simulink model "airgk"  (Simulink 8.7)
settings: Solver=ode45  StartTime=0  StopTime=250  RelTol=1e-3
undefined symbols (not defined in the file or in its folder): GM1, x0, xfix
undefined symbols (not defined in the file): AM, GM2
libraries: airlib x1
(part 1 of 2)
settings Model: Creator=kumabhi  LastModifiedBy=kumabhi
settings DataIOCC: LimitDataPoints=off  SignalLoggingSaveFormat=ModelDataLogs  SaveOutput=off  SaveTime=off
settings OptimizationCC: BlockReduction=off  BooleanDataType=off  InitFltsAndDblsToZero=on
settings DebuggingCC: SaveWithParameterizedLinksMsg=none  SignalResolutionControl=TryResolveAllWithWarning  MultiTaskDSMMsg=warning  MultiTaskCondExecSysMsg=none  StrictBusMsg=None
settings HardwareCC: ProdBitPerPointer=64  ProdLargestAtomicFloat=Float  ProdIntDivRoundTo=Zero  ProdEndianess=LittleEndian  ProdWordSize=64  ProdHWDeviceType=Intel->x86-64 (Windows64)  TargetUnknown=on
settings GRTTargetCC: TargetFcnLib=ansi_tfl_tmw.mat  GeneratePreprocessorConditionals=Use local settings  CombineOutputUpdateFcns=off  GRTInterface=on
settings ConfigComp: CovModelRefEnable=off

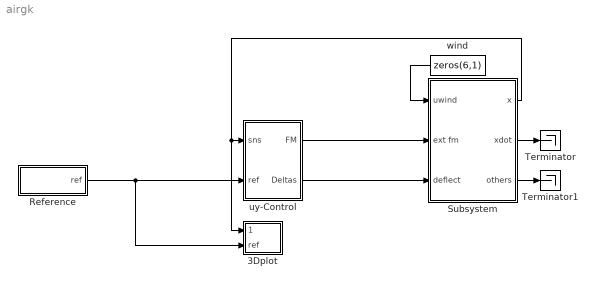
== system airgk ==
  3Dplot : Subsystem
  Reference : Subsystem  mask(Reference Path Generation){Px=[0          2000          2000             0             0             0], Py=[0             0          2000          2000          1000             0], Ph=[60           100            60           500            60            60], Pt=[0   33.3400   66.6800  100.8105  119.0191  135.6858], T=0.05}
      mask prompts: Px "X Positions"; Py "Y Positions"; Ph "H Positions"; Pt "Time"; T "Sample Time"
      mask help: This block generates a 3D trajectory. The output is a vector containing the position and velocity of a point that sequentially visits each X,Y,Z position at the corresponding time. The velocity is constant between one visited point and the next.
      mask Help: This block generates a 3D trajectory. The output is a vector containing the position and velocity of a point that sequentially visits each X,Y,Z position at the corresponding time. The velocity is constant between one visited point and the next.
  Subsystem : Subsystem
  Terminator : Terminator
  Terminator1 : Terminator
  uy-Control : Subsystem  mask(General Nonlinear Aircraft Controller){GM1=[0.5486  5.1511  2.8261   47.2259  90.9483  111.4754   0  -6.6462  0   190.512], CD_wind=[0.060  0.430  0  0.0180  0], CL_wind=[0.385  4.78  8.05  0.401  0], Cm_body=[0.194  -2.12   -36.6   -1.76    0], Cl_body=[0   -0.023   -0.450   0.265   -0.161  -0.00229], Cn_body=[0    0.109  -0.110  -0.200    0.0200  -0.0917], K=[-6.75 9 -9 13.5 0.3], THor=15, Ts=0.05}
      mask prompts: GM1 "Geometry and Mass : [cbar   b    S    Ix   Iy   Iz   Jxy  Jxz  Jyz  m]"; CD_wind "Aerodynamic D-Force Derivatives : [CD0 CDa CDq CDde CDih]"; CL_wind "Aerodynamic L-Force Derivatives : [CL0 CLa CLq CLde CLih]"; Cm_body "Aerodynamic Y-Moment Derivatives : [Cm0 Cma Cmq Cmde Cmih]"; Cl_body "Aerodynamic X-moment Derivatives : [Cl0 Clb Clp Clr Clda Cldr]"; Cn_body "Aerodynamic Z-moment Derivatives : [Cn0 Cnb Cnp Cnr Cnda Cndr]"; K "Controller Coefficients: [Ka Kb Kc Kd Ku]"; THor "Horizon Time"; Ts "Sampling Time"
      mask help:
      | This block is a general feedback linearization controller for aircraft.
      | The first input is a vector contains the 12 aircraft states.
      | The second input contains the reference position and velocity.
      | The output contains the commanded deflections (elevator, aileron and rudder) and the thrust force along the body x axis. Geometry, Mass and Aerodynamic Derivatives should match the ones of the aircraft to be controlled. Ka,Kb,Kc,Kd, are the state space (scalar) coefficients of a PID controller for the feedback linearized attitude dynamics, which behaves as a double integrator system. Ku is the proportional forward velocity controller. The Horizon time is the approximated time lag between reference and actual trajectory. Usually only the aircraft related coefficients need to be changed when applying the controller to a different aircraft.
      mask Help:
      | <p>
      |   This block is a general feedback linearization controller for aircraft.
      |   The first input is a vector contains the 12 aircraft states.
      |   The second input contains the reference position and velocity.
      |   The output contains the commanded deflections (elevator,
      |   aileron and rudder) and the thrust force along the body x axis.
      |   Geometry, Mass and Aerodynamic Derivatives should match the
      |   ones of the aircraft to be controlled. Ka,Kb,Kc,Kd, are the state space
      |   (scalar) coefficients of a PID controller for the feedback linearized
      |   attitude dynamics, which behaves as a double integrator system.
      |   Ku is the proportional forward velocity controller. The Horizon time
      |   is the approximated time lag between reference and actual trajectory.
      |   Usually only the aircraft related coefficients need to be changed
      |   when applying the controller to a different aircraft.
      | </p>
      | <p>
      | Note that neither flaps nor stabilators can be used by this control. Also, this control can be used only when the linearized system having thrust, elevators, ailerons, rudder as inputs, and speed, roll, pitch, yaw as outputs is non-minimum phase. Usually such a system has 2 zeros on the negative real axis, related to alpha and beta respectively. Only occasionally the zero related to beta is on the positive real axis. In those cases the system is non-minimum phase and this controller is not usable anymore.
      | </p>
      | <p>
      | The control surface sign conventions are the same adopted in books such as Stevens-Lewis and Etkin, and in many flight simulators,
      | including the FDC toolbox. <br>
      | Specifically, positive elevator deflection causes negative pitching moment (Cmde &#60 0), positive rudder deflection causes negative yawing
      | moment (Cndr &#60 0), and positive aileron deflection causes negative rolling moment (Clda &#60 0). Another way to say the same thing is
      | that, the positive elevators deflection is Trailing Edge Down (TED), the positive rudder(s) deflection is Trailing Edge Left (TEL), and,
      | taking as TED the positive ailerons deflection, da=K*(da_right-da_left), with K usually equal to 1 (FDC) or 1/2.
      | </p>
      | <p>
      | Since this block is largely based on the FDC toolbox, i redirect you to the FDC Toolbox manual, for a good explanation of the underlying
      | components. Besides the mask and the fact that the aerodynamic derivatives are expressed in the stability axis, the only relevant difference
      | with the FDC toolbox is that in the computation of the aerodynamic forces, q is normalized as q*cbar/2V instead of q*cbar/V. The majority
      | of aeronautics books that i've seen use q*cbar/2V.
      | </p>
      | <p>
      | Please note that the International Measurement System is adopted. So, lengths are in meters, masses in Kg, and inertia moments in Kg*m^2.
      | Moreover, forces are in N, moments in N*m, accelerations in g, and angles in radians. For those that use the english system, here are some useful
      | conversion factors: <br>
      | 1 ft   = 0.3048 m, 1 lb   = 0.4536 Kg, 1 slug = 14.593903 Kg ,  1 slug*ft^2 = 1.355818 Kg*m^2
      | <br>
      | </p>
      | <p>
      | Finally, there is an <A HREF="http://www.aae.uiuc.edu/m-selig/apasim/Aircraft-uiuc.html">excellent source</A> of aircraft aerodynamic data
      | which is mantained by Michael S. Selig, Rob Deters, and Glen Dimock at the university of Urbana-Champaign. To use any of the given models
      | you just need to type the supplied aircraft data in the block mask.
      | </p>
      | <p>
      | <p>
      | July 2006, Giampiero Campa
      | </p>
      | </p>
      mask Display: disp('General\nAircraft\nController')
  wind : Constant  Value=zeros(6,1)
  wires:
  wind/1 -> Subsystem/1(" uwind")
  Reference/1(ref) -> uy-Control/2(ref), 3Dplot/2(ref)
  uy-Control/1(FM) -> Subsystem/2(ext fm)
  uy-Control/2(Deltas) -> Subsystem/3(deflect)
  Subsystem/1(x) -> 3Dplot/1(meas), uy-Control/1(sns)
  Subsystem/2(xdot) -> Terminator/1
  Subsystem/3(others) -> Terminator1/1

== system airgk/3Dplot ==
  note: Set Camera position to [0 0 1] for 2D view
  meas : Inport
  ref : Inport  Port=2
  3D Graph : S-Function  LoadFcn=if exist('sfun3d','file'), sfun3d([],[],[],'LoadBlock'); end  FunctionName=sfun3d  Parameters=ax,T,np,cp,gd,ls,mk,mx,hd,tb  SFunctionDeploymentMode=off  EnableBusSupport=off  mask(3D Graph){np=2, ax=[-1 3 -1 3 0 0.5]*1e3, mx=1e3, T=0.1, cp=[-10 -20 3]*1e3, gd=on, hd=on, tb=off, ls=-, mk=none}
      mask prompts: np "Number of moving points (lines)"; ax "Range: [xmin xmax  ymin ymax zmin zmax]"; mx "Max number of points in each line"; T "Sampling Time"; cp "Camera position (use [0 0 1] for 2D XY view)"; gd "Grid (on|off)"; hd "HeadMarkers (on|off)"; tb "Toolbar (on|off)"; ls "LineStyle"; mk "LineMarker"
      mask help:
      | This block plots the position of several points in the XYZ space. The input contains the coordinates of all the points (x1,y1,z1,x2,y2,z2,...).
      | The number of moving points (lines), the XYZ ranges, sampling time, camera position, and grid (among other things) can be set as mask parameters.
      settings: CopyFcn=if exist('sfun3d','file'), sfun3d([],[],[],'CopyBlock'); end  DeleteFcn=if exist('sfun3d','file'), sfun3d([],[],[],'DeleteBlock'); end  NameChangeFcn=if exist('sfun3d','file'), sfun3d([],[],[],'NameChange'); end
      mask Help:
      | This block plots the position of several points in the XYZ space. The input contains the coordinates of all the points (x1,y1,z1,x2,y2,z2,...).
      | The number of moving points (lines), the XYZ ranges, sampling time, camera position, and grid (among other things) can be set as mask parameters.
      mask TypeOptions ls: - | -- | : | -. | none
      mask TypeOptions mk: none | . | + | o | * | x | square | diamond | v | ^ | > | < | pentagram | hexagram
      mask Display: plot([.05 .95 .95 .05 .05],[.45 .45 .95 .95 .45], 0.5+cos(0:0.1:2*pi)*0.3,0.7+sin(0:0.1:2*pi)*0.2)
  Mux3 : Mux  Inputs=[3 3]
  real xyz : Selector  InputPortWidth=12  IndexOptions=Index vector (dialog)  Indices=10:12  OutputSizes=1
  ref xyz : Selector  InputPortWidth=6  IndexOptions=Index vector (dialog)  Indices=1:3  OutputSizes=1
  wires:
  real xyz/1 -> Mux3/1
  ref/1 -> ref xyz/1
  meas/1 -> real xyz/1
  ref xyz/1 -> Mux3/2
  Mux3/1 -> 3D Graph/1

== system airgk/Reference ==
  Clock : Clock
  Delay : UnitDelay  InitialCondition=[Px(1) Py(1) Ph(1)]  SampleTime=T
  Derivative : Subsystem  mask(Time Derivative){x0=[Px(1) Py(1) Ph(1)]'-[Px(2)-Px(1) Py(2)-Py(1) Ph(2)-Ph(1)]'/(Pt(2)-Pt(1))*T, T=T}
      mask prompts: x0 "Initial Condition"; T "Sampling Time"
      mask help:
      | First order approximation of the time derivative of the input signal,
      |   the original one is buggy.
  Hd(t) : Lookup  InputValues=Pt  Table=Ph  SaturateOnIntegerOverflow=on
  Horizon Time : Constant  Value=0
  Math Function : Math  Operator=mod  SaturateOnIntegerOverflow=on
  Mux : Mux  Inputs=3
  Mux2 : Mux  Inputs=[3 3]
  Sum2 : Sum  Inputs=++|  SaturateOnIntegerOverflow=on  InputSameDT=on  OutDataTypeStr=Inherit: Same as first input
  Time Limit : Constant  Value=Pt(end)
  Xd(t) : Lookup  InputValues=Pt  Table=Px  SaturateOnIntegerOverflow=on
  Yd(t) : Lookup  InputValues=Pt  Table=Py  SaturateOnIntegerOverflow=on
  ref : Outport
  wires:
  Mux/1 -> Derivative/1(x), Delay/1
  Time Limit/1 -> Math Function/2
  Math Function/1 -> Hd(t)/1, Yd(t)/1, Xd(t)/1
  Clock/1 -> Sum2/2
  Horizon Time/1 -> Sum2/1
  Sum2/1 -> Math Function/1
  Hd(t)/1 -> Mux/3
  Yd(t)/1 -> Mux/2
  Xd(t)/1 -> Mux/1
  Delay/1 -> Mux2/1
  Derivative/1(xdot) -> Mux2/2
  Mux2/1 -> ref/1

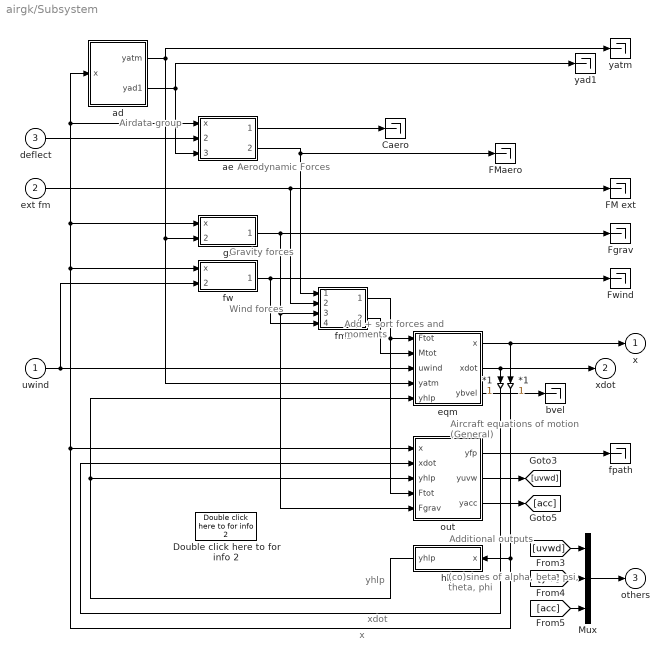
== system airgk/Subsystem ==
  note: xdot
  note: x
  note: yhlp
  note: Additional outputs
  note: Aircraft equations
      | of motion (General)
  note: Wind forces
  note: Gravity forces
  note: Aerodynamic
      | Forces
  note: (co)sines of
      | alpha, beta,
      | psi, theta, phi
  note: Add + sort
      | forces and
      | moments
  note: Airdata group
  " uwind" : Inport
  ext fm : Inport  Port=2
  deflect : Inport  Port=3
  " *1" : Gain  SaturateOnIntegerOverflow=on  OutDataTypeStr=Inherit: Same as input  ParamDataTypeStr=Inherit: Same as input
  *1 : Gain  SaturateOnIntegerOverflow=on  OutDataTypeStr=Inherit: Same as input  ParamDataTypeStr=Inherit: Same as input
  Caero : Terminator
  Double click here to for info 2 : airlib/DT-B747/Double click here to for info 2  SystemSampleTime=-1
  FM ext : Terminator
  FMaero : Terminator
  Fgrav : Terminator
  Fwind : Terminator
  Mux : Mux  Inputs=[3 3 6]
  ad : Subsystem
  ae : Subsystem
  bvel : Terminator
  eqm : Subsystem
  fms : Subsystem  mask(FMsort){}
      mask help: Forces and Moments sorting block
      mask Display: disp('FMsort')
  fpath : Terminator
  fw : Subsystem  mask(fwind){m=GM1(10)}
      mask prompts: m "Mass of the aircraft [kg]:"
      mask help: Forces due to non-steady atmosphere.
      mask Display: disp('Fwind')
  gr : Subsystem  mask(Gravity){m=GM1(10)}
      mask prompts: m "Mass of the aircraft [kg]:"
      mask help: Gravity forces.
      mask Display: disp('Gravity')
  hlp : Subsystem  mask(Hlpfcn){}
      mask help: Help sines and cosines
      mask Display: disp('hlpfcn')
  out : Subsystem
  yad1 : Terminator
  yatm : Terminator
  x : Outport
  xdot : Outport  Port=2
  others : Outport  Port=3
  wires:
  fms/1(Ftot) -> out/4(Ftot), eqm/1(Ftot)
  ext fm/1 -> fms/2(FMprop), FM ext/1
  deflect/1 -> ae/2(uaero)
  ae/1(Caero) -> Caero/1
  eqm/3(ybvel) -> bvel/1
  out/1(yfp) -> fpath/1
  ad/2(yad1) -> yad1/1, ae/3(yad1)
  ad/1(yatm) -> yatm/1, eqm/4(yatm), gr/2(yatm)
  out/3(yacc) -> [acc]
  fw/1(Fwind) -> Fwind/1, fms/4(Fwind)
  ae/2(FMaero) -> FMaero/1, fms/1(FMaero)
  hlp/1(yhlp) -> eqm/5(yhlp), out/3(yhlp)
  " uwind"/1 -> eqm/3(uwind), fw/2(uwind)
  *1/1 -> out/2(xdot)
  gr/1(Fgrav) -> fms/3(Fgrav), out/5(Fgrav), Fgrav/1
  " *1"/1 -> hlp/1(x), out/1(x), fw/1(x), gr/1(x), ae/1(x), ad/1(x)
  eqm/2(xdot) -> xdot/1, *1/1
  eqm/1(x) -> x/1, " *1"/1
  fms/2(Mtot) -> eqm/2(Mtot)
  out/2(yuvw) -> [uvwd]
  [uvwd] -> Mux/1
  [ydl] -> Mux/2
  [acc] -> Mux/3
  Mux/1 -> others/1

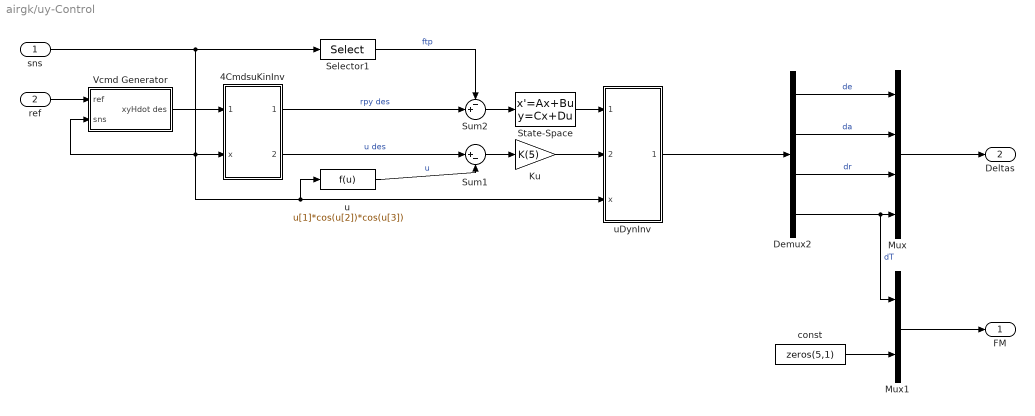
== system airgk/uy-Control ==
  sns : Inport
  ref : Inport  Port=2
  4CmdsuKinInv : Subsystem  mask(Inverse Nonlinear Aircraft Model){Psi0=0, T=Ts}
      mask prompts: Psi0 "Initial Psi (used for Turn Coordination Derivative)"; T "Sampling Time (used for Turn Coordination Derivative)"
      mask help:
      | This block uses an exact turn coordination constraint
      |   to obtain velocity and attitude commands from desired accelerations.
      |   The first input contains the desired derivatives of the position (x,y,H).
      |   The second input contains the actual state of the aircraft.
      |   The first and second outputs contain respectively the commanded
      |   euler angles and the speed along the x axis (u=Vcos(a)cos(b)).
      |   NB : The International measurement system (MKS) is adopted.
      mask Help:
      | This block uses an exact turn coordination constraint
      |   to obtain velocity and attitude commands from desired accelerations.
      |   The first input contains the desired derivatives of the position (x,y,H).
      |   The second input contains the actual state of the aircraft.
      |   The first and second outputs contain respectively the commanded
      |   euler angles and the speed along the x axis (u=Vcos(a)cos(b)).
      |   NB : The International measurement system (MKS) is adopted.
      mask Display: disp('u-Inverse\nKinematic\nModel')
  Demux2 : Demux
  Ku : Gain  Gain=K(5)  SaturateOnIntegerOverflow=on  OutDataTypeStr=Inherit: Same as input  ParamDataTypeStr=Inherit: Same as input
  Mux : Mux  Inputs=[1 1 1 1]
  Mux1 : Mux  Inputs=[1 5]
  Selector1 : Selector  InputPortWidth=12  IndexOptions=Index vector (dialog)  Indices=[9 8 7]  OutputSizes=1
  State-Space : StateSpace  A=K(1)*eye(3)  B=K(2)*eye(3)  C=K(3)*eye(3)  D=K(4)*eye(3)  X0=0
  Sum1 : Sum  Inputs=|+-  SaturateOnIntegerOverflow=on  InputSameDT=on  OutDataTypeStr=Inherit: Same as first input
  Sum2 : Sum  Inputs=-+|  SaturateOnIntegerOverflow=on  InputSameDT=on  OutDataTypeStr=Inherit: Same as first input
  Vcmd Generator : Subsystem  mask(Velocity Command Generator){Kp=1, Kv=0, THor=THor, T=Ts}
      mask prompts: Kp "Position Error Gain"; Kv "Velocity Error Gain"; THor "Horizon Time"; T "Sample Time"
      mask help:
      | The first input is a reference position and velocity vector,
      |   the second one is a current position and velocity vector.
      |   The output is a filtered command in xyHdot .
      mask Help:
      | The first input is a reference position and velocity vector,
      |   the second one is a current position and velocity vector.
      |   The output is a filtered command in xyHdot .
  const : Constant  Value=zeros(5,1)
  u : Fcn  Expr=u[1]*cos(u[2])*cos(u[3])
  uDynInv : Subsystem  mask(Inverse Nonlinear Aircraft Model){GM1=GM1, CD_wind=CD_wind, CL_wind=CL_wind, Cm_body=Cm_body, Cl_body=Cl_body, Cn_body=Cn_body}
      mask prompts: GM1 "Geometry, Mass : [cbar   b    S    Ix   Iy   Iz   Jxy  Jxz  Jyz  m]"; CD_wind "Aerodynamic D-Force Derivatives : [CD0 CDa CDq CDde CDih]"; CL_wind "Aerodynamic L-Force Derivatives : [CL0 CLa CLq CLde CLih]"; Cm_body "Aerodynamic Y-Moment Derivatives : [Cm0 Cma Cmq Cmde Cmih]"; Cl_body "Aerodynamic X-moment Derivatives : [Cl0 Clb Clp Clr Clda Cldr]"; Cn_body "Aerodynamic Z-moment Derivatives : [Cn0 Cnb Cnp Cnr Cnda Cndr]"
      mask help:
      | The first and second inputs contain the desired double derivatives
      |   of the attitude (roll, pitch, and yaw) and the desired detivative of
      |   u=V*cos(alpha)*cos(beta), which is the speed along the x body axis.
      |   The third input contains the actual state of the aircraft.
      |   The output contains the commanded deflections (elevator,
      |   aileron and rudder) and thrust force along the body x axis.
      |   NB : The International measurement system (MKS) is adopted.
      mask init:
      | AM=zeros(6,19);
      | AM(1,[1 2 9 11 12])=reshape(CD_wind,1,5);
      | AM(3,[1 2 9 11 12])=reshape(CL_wind,1,5);
      | AM(5,[1 2 9 11 12])=reshape(Cm_body,1,5);
      | AM(4,[1 5 8 10 13 14])=reshape(Cl_body,1,6);
      | AM(6,[1 5 8 10 13 14])=reshape(Cn_body,1,6);
      | 
      | Ix=GM1(4);Iy=GM1(5);Iz=GM1(6);
      | Jxy=GM1(7);Jxz=GM1(8);Jyz=GM1(9);
      | 
      | detI = Ix*Iy*Iz - 2*Jxy*Jxz*Jyz - Ix*Jyz^2 - Iy*Jxz^2 - Iz*Jxy^2;
      | I1   = Iy*Iz - Jyz^2;I2   = Jxy*Iz + Jyz*Jxz;
      | I3   = Jxy*Jyz + Iy*Jxz;I4   = Ix*Iz - Jxz^2;
      | I5   = Ix*Jyz + Jxy*Jxz;I6   = Ix*Iy - Jxy^2;
      | 
      | Pl  = I1/detI; Pm = I2/detI; Pn = I3/detI;
      | Ppp = -(Jxz*I2 - Jxy*I3)/detI;Ppq = (Jxz*I1 - Jyz*I2 - (Iy-Ix)*I3)/detI;
      | Ppr = -(Jxy*I1 + (Ix-Iz)*I2 - Jyz*I3)/detI;Pqq = (Jyz*I1 - Jxy*I3)/detI;
      | Pqr = -((Iz-Iy)*I1 - Jxy*I2 + Jxz*I3)/detI;Prr = -(Jyz*I1 - Jxz*I2)/detI;
      | 
      | Ql  = I2/detI; Qm = I4/detI; Qn = I5/detI;
      | Qpp = -(Jxz*I4 - Jxy*I5)/detI;Qpq = (Jxz*I2 - Jyz*I4 - (Iy-Ix)*I5)/detI;
      | Qpr = -(Jxy*I2 + (Ix-Iz)*I4 - Jyz*I5)/detI;Qqq = (Jyz*I2 - Jxy*I5)/detI;
      | Qqr = -((Iz-Iy)*I2 - Jxy*I4 + Jxz*I5)/detI;Qrr = -(Jyz*I2 - Jxz*I4)/detI;
      | 
      | Rl  = I3/detI; Rm = I5/detI; Rn = I6/detI;
      | Rpp = -(Jxz*I5 - Jxy*I6)/detI;
      | Rpq = (Jxz*I3 - Jyz*I5 - (Iy-Ix)*I6)/detI;
      | Rpr = -(Jxy*I3 + (Ix-Iz)*I5 - Jyz*I6)/detI;
      | Rqq = (Jyz*I3 - Jxy*I6)/detI;
      | Rqr = -((Iz-Iy)*I3 - Jxy*I5 + Jxz*I6)/detI;
      | Rrr = -(Jyz*I3 - Jxz*I5)/detI;
      | 
      | GM2 = [  Pl   Pm   Pn   Ppp  Ppq  Ppr  Pqq  Pqr  Prr ;
      |                Ql  Qm   Qn   Qpp  Qpq  Qpr  Qqq  Qqr  Qrr ;
      |                Rl  Rm   Rn   Rpp  Rpq  Rpr  Rqq  Rqr  Rrr ];
      | 
      | xfix=1;
      mask Help:
      | <p>
      | This block is an inverse nonlinear 6DOF aircraft model, with a very accurate built-in atmosphere model and constant aerodynamic derivatives.
      | The architecture of the block is largely based on the Aircraft block provided by the <A
      | HREF="http://www.mathworks.com/matlabcentral/fileexchange/loadFile.do?objectId=252&objectType=file">FDC toolbox</A> (Marc Rauw, 1993-2000).
      | </p>
      | <p>
      | The geometric and inertal data of the aircraft are entered as parameters in the first row of the mask, sampling time is the last parameter. The other rows contain the non-dimensional aerodynamic derivatives.
      | </p>
      | <p>
      |   The first and second inputs contain the desired double derivatives
      |   of the attitude (roll, pitch, and yaw) and the desired detivative of
      |   u=V*cos(alpha)*cos(beta), which is the speed along the x body axis.
      |   The third input contains the actual state of the aircraft.
      |   The output contains the commanded deflections (elevator,
      |   aileron and rudder) and thrust force along the body x axis.
      | </p>
      | <p>
      | Note that neither flaps nor stabilators can be used by this control.
      | </p>
      | <p>
      | The control surface sign conventions are the same adopted in books such as Stevens-Lewis and Etkin, and in many flight simulators,
      | including the FDC toolbox. <br>
      | Specifically, positive elevator deflection causes negative pitching moment (Cmde &#60 0), positive rudder deflection causes negative yawing
      | moment (Cndr &#60 0), and positive aileron deflection causes negative rolling moment (Clda &#60 0). Another way to say the same thing is
      | that, the positive elevators deflection is Trailing Edge Down (TED), the positive rudder(s) deflection is Trailing Edge Left (TEL), and,
      | taking as TED the positive ailerons deflection, da=K*(da_right-da_left), with K usually equal to 1 (FDC) or 1/2.
      | </p>
      | <p>
      | Since this block is largely based on the FDC toolbox, i redirect you to the FDC Toolbox manual, for a good explanation of the underlying
      | components. Besides the mask and the fact that the aerodynamic derivatives are expressed in the stability axis, the only relevant difference
      | with the FDC toolbox is that in the computation of the aerodynamic forces, q is normalized as q*cbar/2V instead of q*cbar/V. The majority
      | of aeronautics books that i've seen use q*cbar/2V.
      | </p>
      | <p>
      | Please note that the International Measurement System is adopted. So, lengths are in meters, masses in Kg, and inertia moments in Kg*m^2.
      | Moreover, forces are in N, moments in N*m, accelerations in g, and angles in radians. For those that still use the english system, here are some useful
      | conversion factors: <br>
      | 1 ft   = 0.3048 m, 1 lb   = 0.4536 Kg, 1 slug = 14.593903 Kg ,  1 slug*ft^2 = 1.355818 Kg*m^2
      | <br>
      | </p>
      | <p>
      | Finally, there is an <A HREF="http://www.aae.uiuc.edu/m-selig/apasim/Aircraft-uiuc.html">excellent source</A> of aircraft aerodynamic data
      | which is mantained by Michael S. Selig, Rob Deters, and Glen Dimock at the university of Urbana-Champaign. To use any of the given models
      | you just need to type the supplied aircraft data in the block mask.
      | </p>
      | <p>
      | <p>
      | Feb 2004, Giampiero Campa
      | </p>
      | </p>
      mask Display: disp('4 Cmds\nu-Inverse\nAircraft\nModel')
  FM : Outport
  Deltas : Outport  Port=2
  wires:
  ref/1 -> Vcmd Generator/1(ref)
  Vcmd Generator/1(xyHdot des) -> 4CmdsuKinInv/1(pdotdes)
  Sum2/1 -> State-Space/1
  Ku/1 -> uDynInv/2(udotdes)
  State-Space/1 -> uDynInv/1(ftpddotdes)
  sns/1 -> Selector1/1, 4CmdsuKinInv/2(x), Vcmd Generator/2(sns), u/1, uDynInv/3(x)
  Selector1/1 -> Sum2/1  "ftp"
  4CmdsuKinInv/1(rpycmd) -> Sum2/2  "rpy des"
  4CmdsuKinInv/2(ucmd) -> Sum1/1  "u des"
  u/1 -> Sum1/2  "u"
  Sum1/1 -> Ku/1
  Mux/1 -> Deltas/1
  Mux1/1 -> FM/1
  const/1 -> Mux1/2
  Demux2/4 -> Mux1/1, Mux/4  "dT"
  Demux2/3 -> Mux/3  "dr"
  Demux2/2 -> Mux/2  "da"
  Demux2/1 -> Mux/1  "de"
  uDynInv/1(Cmds) -> Demux2/1

== system airgk/Reference/Derivative ==
  x : Inport
  Product2 : Product  Inputs=/*  SaturateOnIntegerOverflow=on  RndMeth=Zero  InputSameDT=on  OutDataTypeStr=Inherit: Same as first input
  Sum4 : Sum  Inputs=|+-  SaturateOnIntegerOverflow=on  InputSameDT=on  OutDataTypeStr=Inherit: Same as first input
  Unit Delay1 : UnitDelay  InitialCondition=x0  SampleTime=T
  Zero-Order Hold1 : ZeroOrderHold  SampleTime=T
  m : Constant  Value=T
  xdot : Outport
  wires:
  Sum4/1 -> Product2/2
  Unit Delay1/1 -> Sum4/2
  Zero-Order Hold1/1 -> Sum4/1, Unit Delay1/1
  m/1 -> Product2/1
  Product2/1 -> xdot/1
  x/1 -> Zero-Order Hold1/1

== system airgk/Subsystem/ad ==
  x : Inport
  ad1 : Subsystem  mask(Airdata1){}
      mask help: Basic airdata variables
      mask Display: disp('Airdata1')
  atm : Subsystem  mask(Atmosph){}
      mask help: Atmosphere variables
      mask Display: disp('Atmosph')
  yatm : Outport
  yad1 : Outport  Port=2
  wires:
  x/1 -> atm/1(x), ad1/1(x)
  atm/1(yatm) -> ad1/2(yatm), yatm/1
  ad1/1(yad1) -> yad1/1

== system airgk/Subsystem/ae ==
  x : Inport
  uaero : Inport  Port=2
  yad1 : Inport  Port=3
  aero : Subsystem  mask(Aeromod){}
      mask help: Aerodynamic model of the DHC-2 'Beaver'.
      mask Display: disp('Aeromod\n(General)')
  dl : Subsystem  mask(Dimless){cbar=GM1(1), b=GM1(2)}
      mask prompts: cbar "Mean aerodynamic chord [m]:"; b "Wing span [m]:"
      mask help: Dimensionless rotational velocities.
      mask Display: disp('Dimless')
  fmdims : Subsystem  mask(FMdims){cbar=GM1(1), b=GM1(2), S=GM1(3)}
      mask prompts: cbar "Mean aerodynamic chord [m]:"; b "Wing span [m]:"; S "Wing surface [m^2]:"
      mask help:
      | Calculate forces and moments from
      | dimensionless derivatives.
      mask Display: disp('FMdims')
  Caero : Outport
  FMaero : Outport  Port=2
  wires:
  aero/1(Caero) -> Caero/1, fmdims/2(Force / moment derivatives)
  dl/1(ydl) -> aero/3(ydl)
  x/1 -> dl/1(x), aero/1(x)
  uaero/1 -> aero/2(uaero)
  yad1/1 -> fmdims/1(yad1)
  fmdims/1(Forces and moments) -> FMaero/1

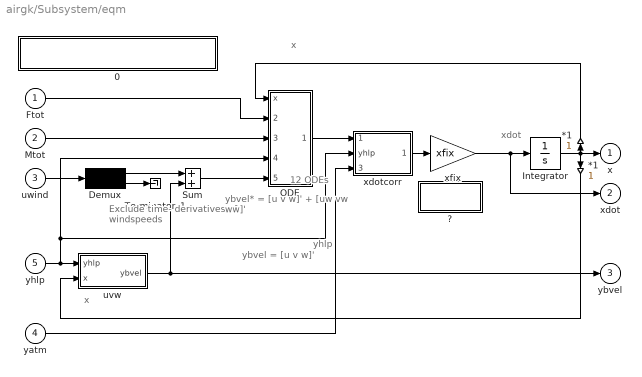
== system airgk/Subsystem/eqm ==
  note: Exclude time-
      | derivatives
      | of windspeeds
  note: ybvel* =
      | [u v w]' +
      | [uw vw ww]'
  note: xdot
  note: x
  note: x
  note: yhlp
  note: ybvel = [u v w]'
  note: 12 ODEs
  Ftot : Inport
  Mtot : Inport  Port=2
  uwind : Inport  Port=3
  yatm : Inport  Port=4
  yhlp : Inport  Port=5
  " *1" : Gain  SaturateOnIntegerOverflow=on  OutDataTypeStr=Inherit: Same as input  ParamDataTypeStr=Inherit: Same as input
  *1 : Gain  SaturateOnIntegerOverflow=on  OutDataTypeStr=Inherit: Same as input  ParamDataTypeStr=Inherit: Same as input
  0 : Subsystem
      mask Display: disp('EQUATIONS OF MOTION (level 3)\nM.O. Rauw')
  "?" : Subsystem
      mask Display: disp('More info\nfor xfix')
  Demux : Demux  Outputs=[3 3]
  Integrator : Integrator  InitialCondition=x0
  ODE : Subsystem
  Sum : Sum  SaturateOnIntegerOverflow=on  InputSameDT=on  OutDataTypeStr=Inherit: Same as first input
  Terminator_1 : Terminator
  uvw : Subsystem  mask(uvw){}
      mask help:
      | Calculation of body-axes velocities
      | u, v, and w
      mask Display: disp('Body-axes\nvelocities')
  xdotcorr : Subsystem  mask(xdotcorr){b=GM1(2), S=GM1(3), m=GM1(10), CYbdot=AM(2,19)}
      mask prompts: b "Wing span [m]:"; S "Wing surface [m^2]:"; m "Mass of the aircraft [kg]:"; CYbdot "Stability-derivative CYbdot:"
      mask help:
      | Correction block to write state
      | equations for DHC-2 Beaver aircraft
      | explicitly.
      mask Display: disp('xdotcorr\n(General)')
  xfix : Gain  Gain=xfix  SaturateOnIntegerOverflow=on  OutDataTypeStr=Inherit: Same as input  ParamDataTypeStr=Inherit: Same as input
  x : Outport
  xdot : Outport  Port=2
  ybvel : Outport  Port=3
  wires:
  Demux/2 -> Terminator_1/1
  yhlp/1 -> uvw/1(yhlp), ODE/4(yhlp), xdotcorr/2(yhlp)
  ODE/1(xdot) -> xdotcorr/1(xdot uncorrected)
  Sum/1 -> ODE/5(ybvel*)
  uvw/1(ybvel) -> ybvel/1, Sum/2
  uwind/1 -> Demux/1
  Demux/1 -> Sum/1
  xdotcorr/1(xdot corrected) -> xfix/1
  yatm/1 -> xdotcorr/3(yatm)
  Ftot/1 -> ODE/2(Ftot)
  Mtot/1 -> ODE/3(Mtot)
  *1/1 -> uvw/2(x)
  Integrator/1 -> x/1, " *1"/1, *1/1
  xfix/1 -> Integrator/1, xdot/1
  " *1"/1 -> ODE/1(x)

== system airgk/Subsystem/fms ==
  FMaero : Inport
  FMprop : Inport  Port=2
  Fgrav : Inport  Port=3
  Fwind : Inport  Port=4
  0 : Subsystem
      mask Display: disp('FMSORT\nM.O. Rauw, October 1997')
  Demux : Demux  Outputs=[3 3]
  Demux1 : Demux  Outputs=[3 3]
  Sum1 : Sum  SaturateOnIntegerOverflow=on  InputSameDT=on  OutDataTypeStr=Inherit: Same as first input
  Sum3 : Sum  Inputs=++++  SaturateOnIntegerOverflow=on  InputSameDT=on  OutDataTypeStr=Inherit: Same as first input
  Ftot : Outport
  Mtot : Outport  Port=2
  wires:
  FMaero/1 -> Demux/1
  FMprop/1 -> Demux1/1
  Demux1/2 -> Sum1/2
  Demux/2 -> Sum1/1
  Fgrav/1 -> Sum3/3
  Demux1/1 -> Sum3/2
  Sum3/1 -> Ftot/1
  Sum1/1 -> Mtot/1
  Demux/1 -> Sum3/1
  Fwind/1 -> Sum3/4

== system airgk/Subsystem/fw ==
  x : Inport
  uwind : Inport  Port=2
  -Xw/m : Fcn  Expr=u[16] + u[5]*u[15] - u[6]*u[14]
  -Yw/m : Fcn  Expr=u[17] - u[4]*u[15] + u[6]*u[13]
  -Zw/m : Fcn  Expr=u[18] + u[4]*u[14] - u[5]*u[13]
  0 : Subsystem
      mask Display: disp('FWIND\nM.O. Rauw, Dec. 1996')
  Mux : Mux  Inputs=3
  Mux1 : Mux  Inputs=[12 6]
  gain : Gain  Gain=-m  SaturateOnIntegerOverflow=on  OutDataTypeStr=Inherit: Same as input  ParamDataTypeStr=Inherit: Same as input
  Fwind : Outport
  wires:
  uwind/1 -> Mux1/2
  x/1 -> Mux1/1
  gain/1 -> Fwind/1
  Mux/1 -> gain/1
  Mux1/1 -> -Yw/m/1, -Zw/m/1, -Xw/m/1
  -Yw/m/1 -> Mux/2
  -Xw/m/1 -> Mux/1
  -Zw/m/1 -> Mux/3

== system airgk/Subsystem/gr ==
  x : Inport
  yatm : Inport  Port=2
  0 : Subsystem
      mask Display: disp('GRAVITY\nM.O. Rauw, October 1997')
  Mux : Mux  Inputs=3
  Mux1 : Mux  Inputs=[12 5]
  Xgr : Fcn  Expr=-m*u[17]*sin(u[8])
  Ygr : Fcn  Expr=m*u[17]*cos(u[8])*sin(u[9])
  Zgr : Fcn  Expr=m*u[17]*cos(u[8])*cos(u[9])
  Fgrav : Outport
  wires:
  Xgr/1 -> Mux/1
  Ygr/1 -> Mux/2
  Mux/1 -> Fgrav/1
  Mux1/1 -> Ygr/1, Xgr/1, Zgr/1
  Zgr/1 -> Mux/3
  x/1 -> Mux1/1
  yatm/1 -> Mux1/2

== system airgk/Subsystem/hlp ==
  x : Inport
  0 : Subsystem
      mask Display: disp('HELP FUNCTIONS\n(often used sines and cosines)\nM.O. Rauw, October 1997')
  Mux : Mux  Inputs=11
  cos alpha : Fcn  Expr=cos(u[2])
  cos beta : Fcn  Expr=cos(u[3])
  cos phi : Fcn  Expr=cos(u[9])
  cos psi : Fcn  Expr=cos(u[7])
  cos theta : Fcn  Expr=cos(u[8])
  sin alpha : Fcn  Expr=sin(u[2])
  sin beta : Fcn  Expr=sin(u[3])
  sin phi : Fcn  Expr=sin(u[9])
  sin psi : Fcn  Expr=sin(u[7])
  sin theta : Fcn  Expr=sin(u[8])
  tan beta : Fcn  Expr=tan(u[3])
  yhlp : Outport
  wires:
  x/1 -> sin psi/1, sin beta/1, cos beta/1, sin alpha/1, cos alpha/1, tan beta/1, sin theta/1, cos theta/1, sin phi/1, cos phi/1, cos psi/1
  cos alpha/1 -> Mux/1
  sin alpha/1 -> Mux/2
  cos beta/1 -> Mux/3
  sin beta/1 -> Mux/4
  tan beta/1 -> Mux/5
  sin psi/1 -> Mux/6
  cos psi/1 -> Mux/7
  sin theta/1 -> Mux/8
  cos theta/1 -> Mux/9
  sin phi/1 -> Mux/10
  Mux/1 -> yhlp/1
  cos phi/1 -> Mux/11

== system airgk/Subsystem/out ==
  note: Flightpath
      | variables
  note: du/dt, dv/dt, dw/dt
      | (output equations!)
  note: Body-axes accelerations
      | and specific forces
  x : Inport
  xdot : Inport  Port=2
  yhlp : Inport  Port=3
  Ftot : Inport  Port=4
  Fgrav : Inport  Port=5
  0 : Subsystem
      mask Display: disp('Additional outputs (level 3)\nM.O. Rauw')
  accel : Subsystem  mask(accel){m=GM1(10)}
      mask prompts: m "Mass of the aircraft [kg]:"
      mask help:
      | Body axes accelerations and
      | specific forces.
      mask Display: disp('Accel')
  fp : Subsystem  mask(Flpath){alpha0=x0(2)}
      mask prompts: alpha0 "Initial value of angle of attack, alpha0:"
      mask help: Flightpath related parameters.
      mask Display: disp('flpath')
  uvwdot : Subsystem  mask(uvwdot){}
      mask help: Calculation of du/dt, dv/dt, and dw/dt.
      mask Display: disp('uvwdot')
  yfp : Outport
  yuvw : Outport  Port=2
  yacc : Outport  Port=3
  wires:
  fp/1(yfp) -> yfp/1
  uvwdot/1(yuvw =  [udot; vdot; wdot]) -> yuvw/1
  yhlp/1 -> uvwdot/3(yhlp)
  Ftot/1 -> accel/1(Ftot)
  accel/1(yacc) -> yacc/1
  xdot/1 -> fp/2(xdot), uvwdot/2(xdot)
  x/1 -> fp/1(x), uvwdot/1(x)
  Fgrav/1 -> accel/2(Fgrav)

== system airgk/uy-Control/4CmdsuKinInv ==
  pdotdes : Inport
  x : Inport  Port=2
  Demux : Demux  Outputs=3
  Exact Turn Coordination : Subsystem
  Mux1 : Mux  Inputs=3
  Mux2 : Mux  Inputs=[3 12]
  a2c  xy : Subsystem  mask(Continuous Atan2 Function){L=4, T=T}
      mask prompts: L "Maximum angular distance covered during the sample time (< 2*pi)"; T "Sample Time"
      mask help:
      | This atan2 does not jump between pi and -pi.
      |   It is assumed that the inputs changes smoothly in time,
      |   specifically it is assumed that the maximum magnitude of the
      |   angular velocity of the input point [x,y] is less than L/T [rad/sec],
      |   where L and T are the first and second parameters in the mask.
  a2c xz : Subsystem  mask(Continuous Atan2 Function){L=4, T=T}
      mask prompts: L "Maximum angular distance covered during the sample time (< 2*pi)"; T "Sample Time"
      mask help:
      | This atan2 does not jump between pi and -pi.
      |   It is assumed that the inputs changes smoothly in time,
      |   specifically it is assumed that the maximum magnitude of the
      |   angular velocity of the input point [x,y] is less than L/T [rad/sec],
      |   where L and T are the first and second parameters in the mask.
  function : Fcn  Expr=sqrt(abs(u[1]^2+u[2]^2+u[3]^2))*cos(u[3+2])*cos(u[3+3])
  norm Vxy : Fcn  Expr=sqrt(u[1]^2+u[2]^2)
  rpycmd : Outport
  ucmd : Outport  Port=2
  wires:
  x/1 -> Exact Turn Coordination/1(x), Mux2/2
  Exact Turn Coordination/3(psi) -> Mux1/3
  Mux1/1 -> rpycmd/1
  Exact Turn Coordination/2(theta) -> Mux1/2
  Exact Turn Coordination/1(phi) -> Mux1/1
  a2c  xy/1(a) -> Exact Turn Coordination/2(chi)  "chi"
  norm Vxy/1 -> a2c xz/2(x)
  Demux/3 -> a2c xz/1(y)
  Demux/2 -> a2c  xy/1(y)
  Demux/1 -> a2c  xy/2(x)
  a2c xz/1(a) -> Exact Turn Coordination/3(gamma)  "gamma"
  pdotdes/1 -> norm Vxy/1, Mux2/1, Demux/1  "xyHdotdes"
  function/1 -> ucmd/1
  Mux2/1 -> function/1

== system airgk/uy-Control/Vcmd Generator ==
  ref : Inport
  sns : Inport  Port=2
  IIR1 : Subsystem  mask(Discrete Time Second Order IIR){ni=3, w=20/THor, x=1, x0=0, T=T}
      mask prompts: ni "Number of Channels"; w "Poles Magnitude (m)"; x "Poles Damping (x)"; x0 "Initial Condition"; T "Sample Time"
      mask help:
      | Each channel has the transfer function :
      |   1-2*cos(sqrt(1-x^2)*m*T)*exp(-x*m*T)+exp(-2*x*m*T) /
      |   1-2*cos(sqrt(1-x^2)*m*T)*exp(-x*m*T)z^-1+exp(-2*x*m*T)z^-2
      |   which is a good (pz-matched) approximation of
      |   m^2/(s^2+2xms+m^2) if 10*m*T<pi
      |   The initial condition is in discrete time for the whole system.
      mask init:
      | A=[];B=[];C=[];D=[];
      | for i=1:ni,
      | A=[A,zeros(size(A,1),2);zeros(2,size(A,2)),[0 1; -exp(-2*x*w*T) 2*cos(sqrt(1-x^2)*w*T)*exp(-x*w*T)]];
      | B=[B,zeros(size(B,1),1);zeros(2,size(B,2)),[0;1+exp(-2*x*w*T)-2*cos(sqrt(1-x^2)*w*T)*exp(-x*w*T)]];
      | C=[C,zeros(size(C,1),2);zeros(1,size(C,2)),[-exp(-2*x*w*T)  2*cos(sqrt(1-x^2)*w*T)*exp(-x*w*T)]];
      | D=[D,zeros(size(D,1),1);zeros(1,size(D,2)),1+exp(-2*x*w*T)-2*cos(sqrt(1-x^2)*w*T)*exp(-x*w*T)];
      | end
      mask Help:
      | <p>
      |   Each channel has the transfer function :
      |   1-2*cos(sqrt(1-x^2)*m*T)*exp(-x*m*T)+exp(-2*x*m*T) /
      |   1-2*cos(sqrt(1-x^2)*m*T)*exp(-x*m*T)z^-1+exp(-2*x*m*T)z^-2
      |   which is a good (pz-matched) approximation of
      |   m^2/(s^2+2xms+m^2) if 10*m*T<pi
      | </p>
      | <p>
      |   The initial condition is in discrete time for the whole system.
      |    If the input is an m-channel vector u, being u0 at time zero,
      |    then a suitable initial condition is : x0=ones(2,1)*reshape(u0,1,m)
      | </p>
      mask Display: dpoly(w^2, [1 2*x*w w^2],'s')
  IIR2 : Subsystem  mask(Discrete Time Second Order IIR){ni=3, w=20/THor, x=1, x0=0, T=T}
      mask prompts: ni "Number of Channels"; w "Poles Magnitude (m)"; x "Poles Damping (x)"; x0 "Initial Condition"; T "Sample Time"
      mask help:
      | Each channel has the transfer function :
      |   1-2*cos(sqrt(1-x^2)*m*T)*exp(-x*m*T)+exp(-2*x*m*T) /
      |   1-2*cos(sqrt(1-x^2)*m*T)*exp(-x*m*T)z^-1+exp(-2*x*m*T)z^-2
      |   which is a good (pz-matched) approximation of
      |   m^2/(s^2+2xms+m^2) if 10*m*T<pi
      |   The initial condition is in discrete time for the whole system.
      mask init: same as airgk/uy-Control/Vcmd Generator/IIR1
      mask Help:
      | <p>
      |   Each channel has the transfer function :
      |   1-2*cos(sqrt(1-x^2)*m*T)*exp(-x*m*T)+exp(-2*x*m*T) /
      |   1-2*cos(sqrt(1-x^2)*m*T)*exp(-x*m*T)z^-1+exp(-2*x*m*T)z^-2
      |   which is a good (pz-matched) approximation of
      |   m^2/(s^2+2xms+m^2) if 10*m*T<pi
      | </p>
      | <p>
      |   The initial condition is in discrete time for the whole system.
      |    If the input is an m-channel vector u, being u0 at time zero,
      |    then a suitable initial condition is : x0=ones(2,1)*reshape(u0,1,m)
      | </p>
      mask Display: dpoly(w^2, [1 2*x*w w^2],'s')
  Mux : Mux  Inputs=[3 3]
  Pos Gain : Gain  Gain=Kp/THor  SaturateOnIntegerOverflow=on  OutDataTypeStr=Inherit: Same as input  ParamDataTypeStr=Inherit: Same as input
  Selector1 : Selector  InputPortWidth=6  IndexOptions=Index vector (dialog)  Indices=1:6  OutputSizes=1
  Selector2 : Selector  InputPortWidth=12  IndexOptions=Index vector (dialog)  Indices=10:12  OutputSizes=1
  Selector3 : Selector  InputPortWidth=6  IndexOptions=Index vector (dialog)  Indices=4:6  OutputSizes=1
  Selector5 : Selector  InputPortWidth=6  IndexOptions=Index vector (dialog)  Indices=1:3  OutputSizes=1
  Sum1 : Sum  Inputs=|++  SaturateOnIntegerOverflow=on  InputSameDT=on  OutDataTypeStr=Inherit: Same as first input
  Sum3 : Sum  Inputs=|+-  SaturateOnIntegerOverflow=on  InputSameDT=on  OutDataTypeStr=Inherit: Same as first input
  Vel Gain : Gain  Gain=Kv/THor  SaturateOnIntegerOverflow=on  OutDataTypeStr=Inherit: Same as input  ParamDataTypeStr=Inherit: Same as input
  xyHdot : Subsystem  mask(uvw){}
      mask help:
      | Calculation of earth-axes velocities
      | xdot,ydot,Hdot
      mask Display: disp('Earth-axes\nvelocities')
  xyHdot des : Outport
  wires:
  Pos Gain/1 -> Sum1/1
  Vel Gain/1 -> Sum1/2
  Selector3/1 -> Vel Gain/1
  Sum1/1 -> xyHdot des/1
  ref/1 -> Selector1/1
  sns/1 -> Selector2/1, xyHdot/1(x)
  Sum3/1 -> Selector3/1, Selector5/1
  Selector5/1 -> IIR1/1(In)
  IIR1/1(Out) -> IIR2/1(In)
  IIR2/1(Out) -> Pos Gain/1
  Selector1/1 -> Sum3/1
  Selector2/1 -> Mux/1
  xyHdot/1(xyHdot) -> Mux/2
  Mux/1 -> Sum3/2

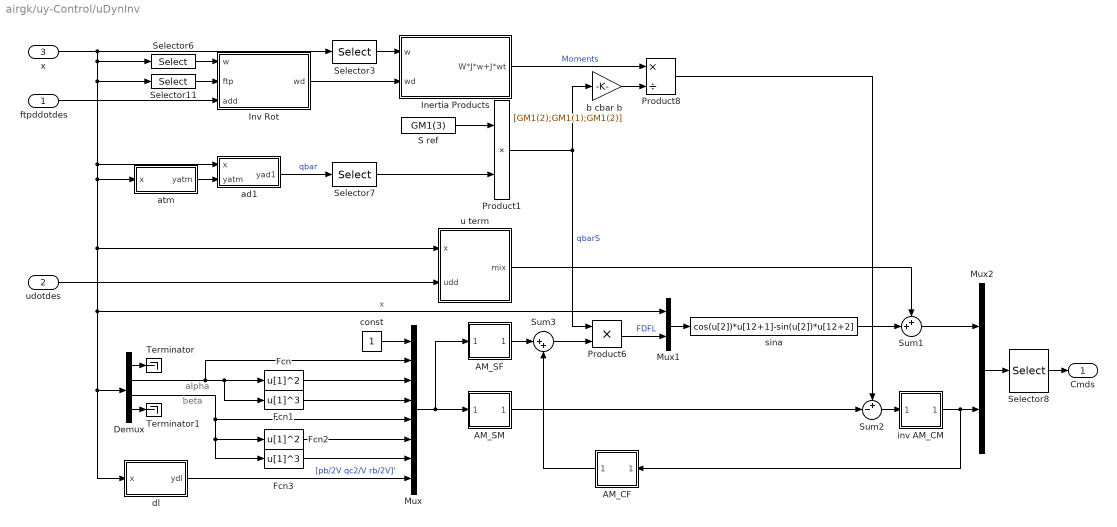
== system airgk/uy-Control/uDynInv ==
  note: beta
  note: alpha
  ftpddotdes : Inport
  udotdes : Inport  Port=2
  x : Inport  Port=3
  " u term" : Subsystem  mask(Vabdot){m=GM1(10)}
      mask prompts: m "Mass of the aircraft [kg]:"
      mask help: Calculation mixed aerodynamic forces
      mask Help: Calculation mixed aerodynamic forces
      mask Display: disp('Mixed\nAerodynamic\nForces')
  AM_CF : Subsystem  mask(State Space){M=AM([1 3],[11 13 14])}
      mask prompts: M "Matrix"
      mask Display: disp('Matrix\nGain')
  AM_SF : Subsystem  mask(State Space){M=AM([1 3],1:10)}
      mask prompts: M "Matrix"
      mask Display: disp('Matrix\nGain')
  AM_SM : Subsystem  mask(State Space){M=AM(4:6,1:10)}
      mask prompts: M "Matrix"
      mask Display: disp('Matrix\nGain')
  Demux : Demux  Outputs=[1 1 1 9]
  Fcn : Fcn  Expr=u[1]^2
  Fcn1 : Fcn  Expr=u[1]^3
  Fcn2 : Fcn  Expr=u[1]^2
  Fcn3 : Fcn  Expr=u[1]^3
  Inertia Products : Subsystem
  Inv Rot : Subsystem
  Mux : Mux  Inputs=[1 1 1 1 1 1 1 3]
  Mux1 : Mux  Inputs=[12 2]
  Mux2 : Mux  Inputs=[1 3]
  Product1 : Product  Inputs=**  SaturateOnIntegerOverflow=on  RndMeth=Zero  InputSameDT=on  OutDataTypeStr=Inherit: Same as first input
  Product6 : Product  Inputs=**  SaturateOnIntegerOverflow=on  RndMeth=Zero  InputSameDT=on  OutDataTypeStr=Inherit: Same as first input
  Product8 : Product  Inputs=*/  SaturateOnIntegerOverflow=on  RndMeth=Zero  InputSameDT=on  OutDataTypeStr=Inherit: Same as first input
  S ref : Constant  Value=GM1(3)
  Selector11 : Selector  InputPortWidth=12  IndexOptions=Index vector (dialog)  Indices=[9 8 7]  OutputSizes=1
  Selector3 : Selector  InputPortWidth=12  IndexOptions=Index vector (dialog)  Indices=[4 5 6]  OutputSizes=1
  Selector6 : Selector  InputPortWidth=12  IndexOptions=Index vector (dialog)  Indices=[4 5 6]  OutputSizes=1
  Selector7 : Selector  InputPortWidth=3  IndexOptions=Index vector (dialog)  Indices=3  OutputSizes=1
  Selector8 : Selector  InputPortWidth=4  IndexOptions=Index vector (dialog)  Indices=[2:4 1]  OutputSizes=1
  Sum1 : Sum  Inputs=++|  SaturateOnIntegerOverflow=on  InputSameDT=on  OutDataTypeStr=Inherit: Same as first input
  Sum2 : Sum  Inputs=+-|  SaturateOnIntegerOverflow=on  InputSameDT=on  OutDataTypeStr=Inherit: Same as first input
  Sum3 : Sum  Inputs=|++  SaturateOnIntegerOverflow=on  InputSameDT=on  OutDataTypeStr=Inherit: Same as first input
  Terminator : Terminator
  Terminator1 : Terminator
  ad1 : Subsystem  mask(Airdata1){}
      mask help: Basic airdata variables
      mask Help: eval('fdchelp airdata1')
      mask Display: disp('Airdata1')
  atm : Subsystem  mask(Atmosph){}
      mask help: Atmosphere variables
      mask Help: eval('fdchelp atmosph')
      mask Display: disp('Atmosph')
  b cbar b : Gain  Gain=[GM1(2);GM1(1);GM1(2)]  SaturateOnIntegerOverflow=on  OutDataTypeStr=Inherit: Same as input  ParamDataTypeStr=Inherit: Same as input
  const : Constant
  dl : Subsystem  mask(Dimless){cbar=GM1(1), b=GM1(2)}
      mask prompts: cbar "Mean aerodynamic chord [m]:"; b "Wing span [m]:"
      mask help: Dimensionless rotational velocities.
      mask Help: eval('fdchelp dimless')
      mask Display: disp('Dimless')
  inv AM_CM : Subsystem  mask(State Space){M=pinv(AM(4:6,[11 13 14]))}
      mask prompts: M "Matrix"
      mask Display: disp('Matrix\nGain')
  sina : Fcn  Expr=cos(u[2])*u[12+1]-sin(u[2])*u[12+2]
  Cmds : Outport
  wires:
  udotdes/1 -> " u term"/2(udd)
  " u term"/1(mix) -> Sum1/1
  Sum1/1 -> Mux2/1
  sina/1 -> Sum1/2
  Selector8/1 -> Cmds/1
  Mux1/1 -> sina/1
  Product6/1 -> Mux1/2  "FDFL"
  Sum3/1 -> Product6/2
  Sum2/1 -> inv AM_CM/1(In1)
  Inertia Products/1(W*J*w+J*wt) -> Product8/1  "Moments"
  Product1/1 -> b cbar b/1, Product6/1  "qbarS"
  b cbar b/1 -> Product8/2
  x/1 -> Selector11/1, " u term"/1(x), Mux1/1, Demux/1, dl/1(x), atm/1(x), ad1/1(x), Selector6/1, Selector3/1  "x"
  Demux/4 -> Terminator1/1
  Demux/1 -> Terminator/1
  const/1 -> Mux/1
  dl/1(ydl) -> Mux/8  "[pb/2V qc2/V rb/2V]'"
  Fcn2/1 -> Mux/6
  Demux/2 -> Fcn1/1, Fcn/1, Mux/2
  Demux/3 -> Fcn3/1, Fcn2/1, Mux/5
  Fcn3/1 -> Mux/7
  Fcn1/1 -> Mux/4
  Fcn/1 -> Mux/3
  Mux/1 -> AM_SM/1(In1), AM_SF/1(In1)
  AM_SM/1(Out1) -> Sum2/2
  AM_SF/1(Out1) -> Sum3/1
  AM_CF/1(Out1) -> Sum3/2
  inv AM_CM/1(Out1) -> AM_CF/1(In1), Mux2/2
  Product8/1 -> Sum2/1
  Mux2/1 -> Selector8/1
  atm/1(yatm) -> ad1/2(yatm)
  ftpddotdes/1 -> Inv Rot/3(add)
  Selector11/1 -> Inv Rot/2(ftp)
  Selector6/1 -> Inv Rot/1(w)
  Inv Rot/1(wd) -> Inertia Products/2(wd)
  S ref/1 -> Product1/1
  Selector3/1 -> Inertia Products/1(w)
  ad1/1(yad1) -> Selector7/1  "qbar"
  Selector7/1 -> Product1/2

== system airgk/Subsystem/ad/ad1 ==
  x : Inport
  yatm : Inport  Port=2
  0 : Subsystem
      mask Display: disp('AIRDATA1\nM.O. Rauw, October 1997')
  M : Fcn  Expr=u[2]/u[1]
  Mux : Mux  Inputs=[1 12]
  Mux1 : Mux  Inputs=[12 5]
  Mux2 : Mux  Inputs=3
  a : Fcn  Expr=sqrt(401.8743*u[3])
  qdyn : Fcn  Expr=0.5*u[13]*u[1]^2
  yad1 : Outport
  wires:
  Mux2/1 -> yad1/1
  qdyn/1 -> Mux2/3
  a/1 -> Mux/1, Mux2/1
  M/1 -> Mux2/2
  Mux1/1 -> qdyn/1
  Mux/1 -> M/1
  x/1 -> Mux/2, Mux1/1
  yatm/1 -> a/1, Mux1/2

== system airgk/Subsystem/ad/atm ==
  x : Inport
  0 : Subsystem
      mask Display: disp('ATMOSPH\nM.O. Rauw, October 1997')
  Mux : Mux  Inputs=2
  Mux1 : Mux  Inputs=[2 1]
  Mux2 : Mux  Inputs=5
  T : Fcn  Expr=288.15 - 0.0065*u[12]
  g : Fcn  Expr=9.80665*(6371020/(6371020+u[12]))^2
  mu : Fcn  Expr=(1.458*10^(-6)*u[2]^1.5)/(u[2]+110.4)
  ps : Fcn  Expr=101325*(u[2]/288.15)^(u[1]/1.86584)
  rho : Fcn  Expr=u[3]/(287.053*u[2])
  yatm : Outport
  wires:
  x/1 -> T/1, g/1
  Mux/1 -> Mux1/1, mu/1, ps/1
  ps/1 -> Mux1/2, Mux2/2
  T/1 -> Mux/2, Mux2/3
  g/1 -> Mux/1, Mux2/5
  rho/1 -> Mux2/1
  Mux1/1 -> rho/1
  Mux2/1 -> yatm/1
  mu/1 -> Mux2/4

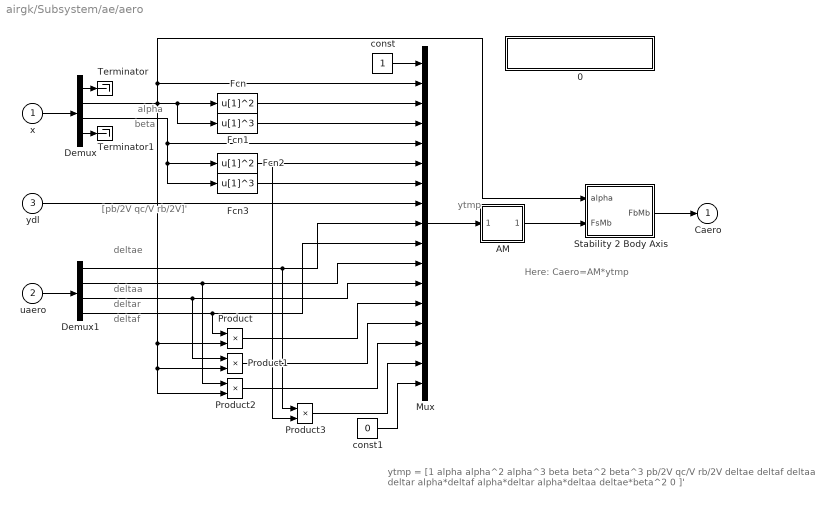
== system airgk/Subsystem/ae/aero ==
  note: ytmp = [1  alpha  alpha^2  alpha^3  beta  beta^2  beta^3  pb/2V  qc/V  rb/2V  deltae
      | deltaf  deltaa  deltar  alpha*deltaf  alpha*deltar  alpha*deltaa  deltae*beta^2  0 ]'
  note: [pb/2V qc/V rb/2V]'
  note: beta
  note: deltae
  note: deltaa
  note: deltar
  note: deltaf
  note: alpha
  note: ytmp
  note: Here: Caero=AM*ytmp
  x : Inport
  uaero : Inport  Port=2
  ydl : Inport  Port=3
  0 : Subsystem
      mask Display: disp('AEROMOD\nM.O. Rauw, October 1997')
  "AM " : Subsystem  mask(State Space){M=AM}
      mask prompts: M "Matrix"
      mask Display: disp('Matrix\nGain')
  Demux : Demux  Outputs=[1 1 1 9]
  Demux1 : Demux
  Fcn : Fcn  Expr=u[1]^2
  Fcn1 : Fcn  Expr=u[1]^3
  Fcn2 : Fcn  Expr=u[1]^2
  Fcn3 : Fcn  Expr=u[1]^3
  Mux : Mux  Inputs=[1 1 1 1 1 1 1 3 1 1 1 1 1 1 1 1 1]
  Product{,1..3} (4 alike) : Product  SaturateOnIntegerOverflow=on  RndMeth=Zero  InputSameDT=on  OutDataTypeStr=Inherit: Same as first input
  Stability 2 Body Axis : Subsystem
  Terminator : Terminator
  Terminator1 : Terminator
  const : Constant
  const1 : Constant  Value=0
  Caero : Outport
  wires:
  Demux/4 -> Terminator1/1
  Demux/1 -> Terminator/1
  const1/1 -> Mux/17
  const/1 -> Mux/1
  ydl/1 -> Mux/8
  Product3/1 -> Mux/16
  Product2/1 -> Mux/15
  Product1/1 -> Mux/14
  Demux1/1 -> Mux/9, Product3/1
  Fcn2/1 -> Mux/6, Product3/2
  Demux1/4 -> Mux/10, Product/1
  Demux/2 -> Fcn/1, Fcn1/1, Product/2, Product1/2, Product2/2, Mux/2, Stability 2 Body Axis/1(alpha)
  Demux/3 -> Mux/5, Fcn2/1, Fcn3/1
  Demux1/2 -> Mux/11, Product2/1
  Demux1/3 -> Mux/12, Product1/1
  Product/1 -> Mux/13
  Fcn3/1 -> Mux/7
  uaero/1 -> Demux1/1
  Fcn1/1 -> Mux/4
  Fcn/1 -> Mux/3
  x/1 -> Demux/1
  Mux/1 -> "AM "/1(In1)
  Stability 2 Body Axis/1(FbMb) -> Caero/1
  "AM "/1(Out1) -> Stability 2 Body Axis/2(FsMb)

== system airgk/Subsystem/ae/dl ==
  x : Inport
  0 : Subsystem
      mask Display: disp('DIMLESS\nM.O. Rauw, October 1997')
  Mux : Mux  Inputs=3
  pb/2V : Fcn  Expr=0.5 * u[4] * b / u[1]
  qc/2V : Fcn  Expr=0.5* u[5] * cbar / u[1]
  rb/2V : Fcn  Expr=0.5 * u[6] * b / u[1]
  ydl : Outport
  wires:
  pb/2V/1 -> Mux/1
  qc/2V/1 -> Mux/2
  rb/2V/1 -> Mux/3
  Mux/1 -> ydl/1
  x/1 -> qc/2V/1, rb/2V/1, pb/2V/1

== system airgk/Subsystem/ae/fmdims ==
  yad1 : Inport
  Force / moment derivatives : Inport  Port=2
  0 : Subsystem
      mask Display: disp('FMDIMS\nM.O. Rauw, October 1997')
  Mux : Mux  Inputs=[3 6]
  Mux1 : Mux  Inputs=6
  S : Gain  Gain=S  SaturateOnIntegerOverflow=on  OutDataTypeStr=Inherit: Same as input  ParamDataTypeStr=Inherit: Same as input
  b : Gain  Gain=b  SaturateOnIntegerOverflow=on  OutDataTypeStr=Inherit: Same as input  ParamDataTypeStr=Inherit: Same as input
  "b " : Gain  Gain=b  SaturateOnIntegerOverflow=on  OutDataTypeStr=Inherit: Same as input  ParamDataTypeStr=Inherit: Same as input
  cbar : Gain  Gain=cbar  SaturateOnIntegerOverflow=on  OutDataTypeStr=Inherit: Same as input  ParamDataTypeStr=Inherit: Same as input
  qdyn * S * CX : Fcn  Expr=u[4]*u[3]
  qdyn * S * CY : Fcn  Expr=u[5]*u[3]
  qdyn * S * CZ : Fcn  Expr=u[6]*u[3]
  qdyn * S * Cl : Fcn  Expr=u[7]*u[3]
  qdyn * S * Cm : Fcn  Expr=u[8]*u[3]
  qdyn * S * Cn : Fcn  Expr=u[9]*u[3]
  Forces and moments : Outport
  wires:
  Mux1/1 -> Forces and moments/1
  "b "/1 -> Mux1/6
  cbar/1 -> Mux1/5
  Force / moment derivatives/1 -> S/1
  Mux/1 -> qdyn * S * CZ/1, qdyn * S * CX/1, qdyn * S * CY/1, qdyn * S * Cl/1, qdyn * S * Cm/1, qdyn * S * Cn/1
  qdyn * S * Cl/1 -> b/1
  qdyn * S * Cm/1 -> cbar/1
  qdyn * S * Cn/1 -> "b "/1
  yad1/1 -> Mux/1
  qdyn * S * CX/1 -> Mux1/1
  qdyn * S * CY/1 -> Mux1/2
  S/1 -> Mux/2
  qdyn * S * CZ/1 -> Mux1/3
  b/1 -> Mux1/4

== system airgk/Subsystem/eqm/0 ==

== system airgk/Subsystem/eqm/? ==

== system airgk/Subsystem/eqm/ODE ==
  x : Inport
  Ftot : Inport  Port=2
  Mtot : Inport  Port=3
  yhlp : Inport  Port=4
  ybvel* : Inport  Port=5
  0 : Subsystem
      mask Display: disp('12 Ordinary Differential\nEquations (level 4)\nM.O. Rauw')
  Eulerdot : Subsystem  mask(Eulerdot){}
      mask help:
      | Calculation of d(psi)/dt, d(theta)/dt,
      | and d(phi/dt)
      mask Display: disp('psi dot\ntheta dot\nphi dot')
  Mux : Mux  Inputs=[12 3 3 11]
  Mux1 : Mux  Inputs=[3 3 3 3]
  Vabdot : Subsystem  mask(Vabdot){m=GM1(10)}
      mask prompts: m "Mass of the aircraft [kg]:"
      mask help: Calculation of dV/dt, dalpha/dt, dbeta/dt.
      mask Display: disp('V dot\nalpha dot\nbeta dot')
  pqrdot : Subsystem  mask(pqrdot){}
      mask help: Calculation of dp/dt, dq/dt, and dr/dt
      mask Display: disp('p dot\nq dot\nr dot')
  xyHdot : Subsystem  mask(xyHdot){}
      mask help: Calculation of d(xe)/dt, d(ye)/dt, and dH/dt
      mask Display: disp('xe dot\nye dot\nH dot')
  xdot : Outport
  wires:
  x/1 -> Mux/1
  Mtot/1 -> Mux/3
  Ftot/1 -> Mux/2
  Mux/1 -> pqrdot/1(upqr), Vabdot/1(uVab), Eulerdot/1(ueul), xyHdot/2(uxYH)
  ybvel*/1 -> xyHdot/1(ybvel*)
  yhlp/1 -> Mux/4
  xyHdot/1(yxyH) -> Mux1/4
  Eulerdot/1(yeul) -> Mux1/3
  pqrdot/1(ypqr) -> Mux1/2
  Vabdot/1(yVab) -> Mux1/1
  Mux1/1 -> xdot/1

== system airgk/Subsystem/eqm/uvw ==
  yhlp : Inport
  x : Inport  Port=2
  0 : Subsystem
      mask Display: disp('UVW\nM.O. Rauw, October 1997')
  Mux : Mux  Inputs=3
  Mux1 : Mux  Inputs=[12 11]
  u : Fcn  Expr=u[1]*u[13]*u[15]
  v : Fcn  Expr=u[1]*u[16]
  w : Fcn  Expr=u[1]*u[14]*u[15]
  ybvel : Outport
  wires:
  Mux1/1 -> v/1, u/1, w/1
  yhlp/1 -> Mux1/2
  x/1 -> Mux1/1
  u/1 -> Mux/1
  v/1 -> Mux/2
  w/1 -> Mux/3
  Mux/1 -> ybvel/1
